simulink model "psm_mpc_ekf_bemf_ctrl"  (R2026a)
settings: Solver=ode23tb  StopTime=simlength  FixedStep=tc  MaxStep=tc
values from neighbouring files (symbols this model uses):
  dead_time_INV = 3e-6    (= 3e-06)    [init_model.m]
  fPWM_INV = fPWM_AFE    (= 15000)    [init_model.m]
  g0_10Hz = fcut_10Hz_flt * ts_afe * 2*pi    (= 0.00418879020479)    [init_model.m]
  g0_1Hz = fcut_1Hz_flt * ts_afe * 2*pi    (= 0.000418879020479)    [init_model.m]
  g1_10Hz = 1 - g0_10Hz    (= 0.995811209795)    [init_model.m]
  g1_1Hz = 1 - g0_1Hz    (= 0.99958112098)    [init_model.m]
  inv_m_scale = motorc_m_scale    [init_model.m]
  iq_lim = 1.4    [init_model.m]
  k_kalman = 0    [init_model.m]
  kg = Kobs(1)    [init_model.m]
  ki_align = 0.1    [init_model.m]
  ki_w = 32    [init_model.m]
  kp_align = 0.6    [init_model.m]
  kp_w = 2    [init_model.m]
  kw = Kobs(2)    [init_model.m]
  lim_down_align = -0.2    [init_model.m]
  lim_up_align = 0.2    [init_model.m]
  number_of_modules = 1    [init_model.m]
  omega_m_sim = omega_m_bez    [init_model.m]
  simlength = 2    [init_model.m]
  tc = ts_afe/100    (= 6.66666666667e-07)    [init_model.m]
  time_gain_afe_module_1 = 1.0    (= 1)    [init_model.m]
  time_gain_inv_module_2 = 1.0    (= 1)    [init_model.m]
  ts_inv = 1/fPWM_INV    (= 6.66666666667e-05)    [init_model.m]
undefined symbols (not defined in the file or in its folder): A1_tilde_ekf, A2_tilde_ekf, A3_tilde_ekf, A4_tilde_ekf, Bd_ekf, C_ekf, ibez, La, Lalpha_norm, Lb, Lbeta_norm, omega_bez, omega_m_bez, psi_bez, psi_m, Qkalman, Rkalman, rpm_base, rpm_bez, Rs, Rs_norm, tau_bez, torque_base, ubez
libraries: fl_lib x24, nesl_utility x11, cstblocks_lti x2, single_phase_pwm_modulator x1, threephase_inductor_lib x1, simple_flexible_shaft x1, permanent_magnet_synchronous_machine x1
(part 2 of 2)

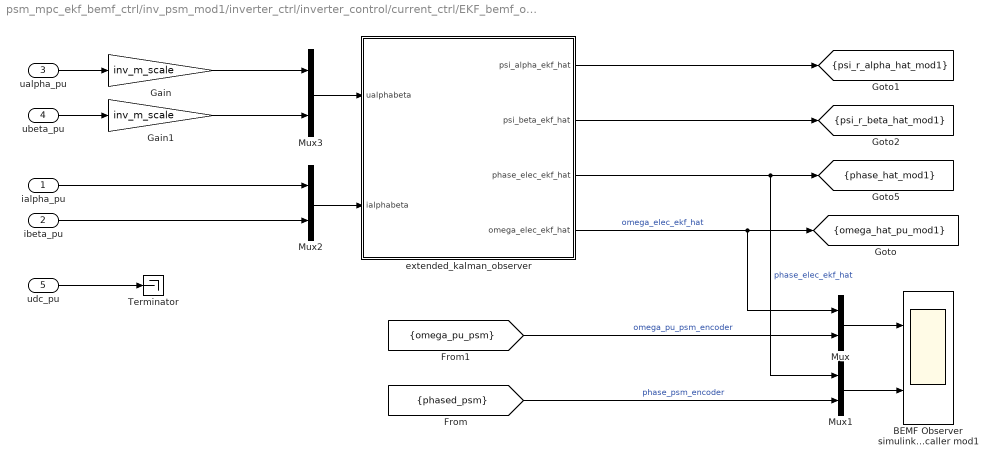
== system psm_mpc_ekf_bemf_ctrl/inv_psm_mod1/inverter_ctrl/inverter_control/current_ctrl/EKF_bemf_observer ==
  ialpha_pu : Inport
  ibeta_pu : Inport  Port=2
  ualpha_pu : Inport  Port=3
  ubeta_pu : Inport  Port=4
  udc_pu : Inport  Port=5
  BEMF Observer simulink/Ccaller mod1 : Scope  NumInputPorts=2
      settings: ActiveDisplayYMinimum=-3.92694091796875  ActiveDisplayYMaximum=3.92645263671875
  Gain : Gain  Gain=inv_m_scale
  Gain1 : Gain  Gain=inv_m_scale
  Mux{,1..3} (4 alike) : Mux  Inputs=2
  Terminator : Terminator
  extended_kalman_observer : Subsystem
  tag scope: omega_hat_pu_mod1=scoped, phase_hat_mod1=scoped, psi_r_alpha_hat_mod1=scoped, psi_r_beta_hat_mod1=scoped
  wires:
  ialpha_pu/1 -> Mux2/1
  ibeta_pu/1 -> Mux2/2
  Mux/1 -> BEMF Observer simulink/Ccaller mod1/1
  Mux1/1 -> BEMF Observer simulink/Ccaller mod1/2
  ualpha_pu/1 -> Gain/1
  ubeta_pu/1 -> Gain1/1
  extended_kalman_observer/3(phase_elec_ekf_hat) -> Mux1/1, [phase_hat_mod1]  "phase_elec_ekf_hat"
  extended_kalman_observer/4(omega_elec_ekf_hat) -> [omega_hat_pu_mod1], Mux/1  "omega_elec_ekf_hat"
  [omega_pu_psm] -> Mux/2  "omega_pu_psm_encoder"
  [phased_psm] -> Mux1/2  "phase_psm_encoder"
  udc_pu/1 -> Terminator/1
  extended_kalman_observer/1(psi_alpha_ekf_hat) -> [psi_r_alpha_hat_mod1]
  extended_kalman_observer/2(psi_beta_ekf_hat) -> [psi_r_beta_hat_mod1]
  Mux2/1 -> extended_kalman_observer/2(ialphabeta)
  Mux3/1 -> extended_kalman_observer/1(ualphabeta)
  Gain/1 -> Mux3/1
  Gain1/1 -> Mux3/2

== system psm_mpc_ekf_bemf_ctrl/inv_psm_mod1/inverter_ctrl/inverter_control/current_ctrl/current_reference_generator ==
  torque_ref_pu : Inport
  theta_elec_hat : Inport  Port=2
  Gain5 : Gain  Gain=-1
  Product : Product
  Product1 : Product
  Trigonometric Function1 : Trigonometry
  Trigonometric Function2 : Trigonometry  Operator=cos
  i_alpha_ref : Outport
  i_beta_ref : Outport  Port=2
  tag scope: ialpha_pu_ref_mod1=scoped, ibeta_pu_ref_mod1=scoped
  wires:
  Trigonometric Function1/1 -> Product/2
  Product1/1 -> [ibeta_pu_ref_mod1], i_beta_ref/1
  Trigonometric Function2/1 -> Product1/2
  Product/1 -> Gain5/1
  Gain5/1 -> [ialpha_pu_ref_mod1], i_alpha_ref/1
  torque_ref_pu/1 -> Product/1, Product1/1
  theta_elec_hat/1 -> Trigonometric Function1/1, Trigonometric Function2/1  "theta_electrical"

== system psm_mpc_ekf_bemf_ctrl/inv_psm_mod1/inverter_ctrl/inverter_control/current_ctrl/current_transformation ==
  Demux : Demux  Outputs=3
  alphabeta2dq : MATLAB Function  TreatAsAtomicUnit=on
  uvw2alphabeta : MATLAB Function  TreatAsAtomicUnit=on
  tag scope: ialpha_pu_mod1=scoped, ibeta_pu_mod1=scoped, id_pu_mod1=scoped, iq_pu_mod1=scoped
  wires:
  alphabeta2dq/2(q) -> [iq_pu_mod1]  "iq_pu"
  alphabeta2dq/1(d) -> [id_pu_mod1]  "id_pu"
  uvw2alphabeta/2(beta) -> alphabeta2dq/2(beta), [ibeta_pu_mod1]  "ibeta_pu"
  uvw2alphabeta/1(alpha) -> [ialpha_pu_mod1], alphabeta2dq/1(alpha)  "ialpha_pu"
  [motor_phase_ctrl_mod1] -> alphabeta2dq/3(gamma)
  Demux/3 -> uvw2alphabeta/3(w)  "iw"
  Demux/2 -> uvw2alphabeta/2(v)  "iv"
  Demux/1 -> uvw2alphabeta/1(u)  "iu"
  [isd_uvw_inv_mod1] -> Demux/1

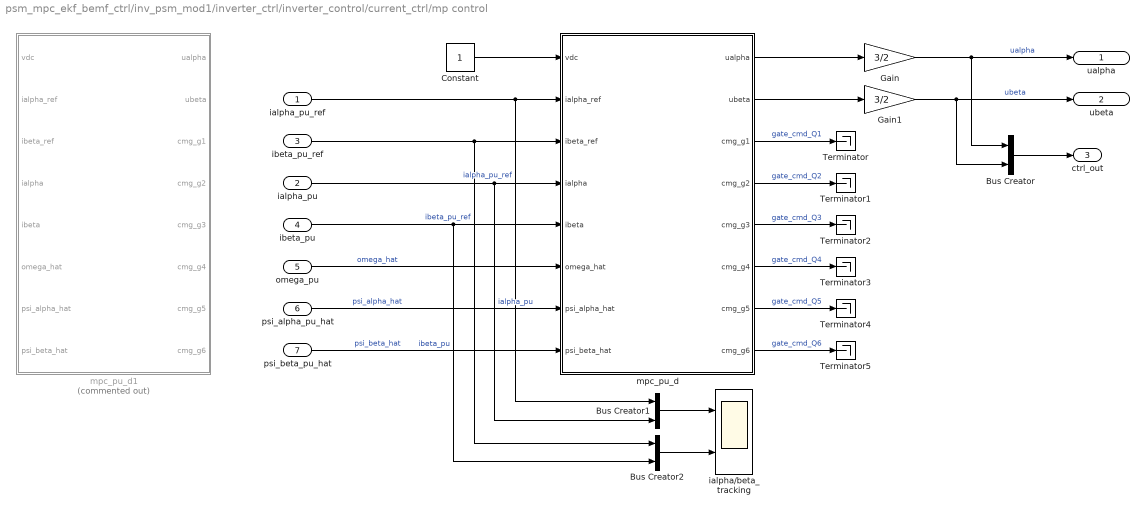
== system psm_mpc_ekf_bemf_ctrl/inv_psm_mod1/inverter_ctrl/inverter_control/current_ctrl/mp control ==
  ialpha_pu_ref : Inport
  ialpha_pu : Inport  Port=2
  ibeta_pu_ref : Inport  Port=3
  ibeta_pu : Inport  Port=4
  omega_pu : Inport  Port=5
  psi_alpha_pu_hat : Inport  Port=6
  psi_beta_pu_hat : Inport  Port=7
  Bus Creator : BusCreator  Inputs=2
  Bus Creator1 : BusCreator  Inputs=2
  Bus Creator2 : BusCreator  Inputs=2
  Constant : Constant
  Gain : Gain  Gain=3/2
  Gain1 : Gain  Gain=3/2
  Terminator{,1..5} (6 alike) : Terminator
  ialpha/beta_tracking : Scope  NumInputPorts=2
      settings: ActiveDisplayYMinimum=-1.13592529296875  ActiveDisplayYMaximum=1.13153076171875  DataLoggingVariableName=ScopeData2
  mpc_pu_d : MATLAB Function  TreatAsAtomicUnit=on
  mpc_pu_d1 : MATLAB Function  Commented=on  TreatAsAtomicUnit=on
  ualpha : Outport
  ubeta : Outport  Port=2
  ctrl_out : Outport  Port=3
  wires:
  ialpha_pu_ref/1 -> mpc_pu_d/2(ialpha_ref), Bus Creator1/1  "ialpha_pu_ref"
  ibeta_pu_ref/1 -> mpc_pu_d/3(ibeta_ref), Bus Creator2/1  "ibeta_pu_ref"
  ialpha_pu/1 -> mpc_pu_d/4(ialpha), Bus Creator1/2  "ialpha_pu"
  ibeta_pu/1 -> mpc_pu_d/5(ibeta), Bus Creator2/2  "ibeta_pu"
  omega_pu/1 -> mpc_pu_d/6(omega_hat)  "omega_hat"
  psi_alpha_pu_hat/1 -> mpc_pu_d/7(psi_alpha_hat)  "psi_alpha_hat"
  psi_beta_pu_hat/1 -> mpc_pu_d/8(psi_beta_hat)  "psi_beta_hat"
  Constant/1 -> mpc_pu_d/1(vdc)
  Bus Creator1/1 -> ialpha/beta_tracking/1
  Bus Creator2/1 -> ialpha/beta_tracking/2
  Bus Creator/1 -> ctrl_out/1
  mpc_pu_d/1(ualpha) -> Gain/1
  mpc_pu_d/2(ubeta) -> Gain1/1
  mpc_pu_d/3(cmg_g1) -> Terminator/1  "gate_cmd_Q1"
  mpc_pu_d/4(cmg_g2) -> Terminator1/1  "gate_cmd_Q2"
  mpc_pu_d/5(cmg_g3) -> Terminator2/1  "gate_cmd_Q3"
  mpc_pu_d/6(cmg_g4) -> Terminator3/1  "gate_cmd_Q4"
  mpc_pu_d/7(cmg_g5) -> Terminator4/1  "gate_cmd_Q5"
  mpc_pu_d/8(cmg_g6) -> Terminator5/1  "gate_cmd_Q6"
  Gain/1 -> Bus Creator/1, ualpha/1  "ualpha"
  Gain1/1 -> Bus Creator/2, ubeta/1  "ubeta"

== system psm_mpc_ekf_bemf_ctrl/inv_psm_mod1/inverter_ctrl/inverter_control/encoder-sensorless-switch/double_integrator_observer ==
  phase_psm : Inport
  Dead Zone : DeadZone  LowerValue=-0.01  UpperValue=0.01
  Gain : Gain  Gain=kw
  Gain1 : Gain  Gain=kg
  Gain2 : Gain  Gain=omega_bez
  Gain3 : Gain  Gain=1/omega_bez
  Gain5 : Gain  Gain=ts_inv
  Sum : Sum  Inputs=-+|
  Sum1 : Sum  Inputs=|++
  Sum2 : Sum  Inputs=|++
  Sum8 : Sum  Inputs=++|
  Unit Delay1 : UnitDelay  InitialCondition=pi  SampleTime=-1
  Unit Delay2 : UnitDelay  SampleTime=-1
  bounder1 : MATLAB Function  TreatAsAtomicUnit=on
  bounder2 : MATLAB Function  TreatAsAtomicUnit=on
  phase_psm_hat : Outport  VectorParamsAs1DForOutWhenUnconnected=off
  omega_pu_psm_hat : Outport  Port=2  VectorParamsAs1DForOutWhenUnconnected=off
  wires:
  Gain1/1 -> Sum2/1
  phase_psm/1 -> Sum/2
  Sum8/1 -> Unit Delay1/1
  Unit Delay1/1 -> bounder2/1(u)
  Sum1/1 -> Unit Delay2/1
  Gain/1 -> Gain3/1
  Unit Delay2/1 -> omega_pu_psm_hat/1, Sum1/2, Gain5/1
  Sum2/1 -> Sum8/2
  bounder2/1(y) -> Sum2/2, phase_psm_hat/1, Sum/1  "phase_hat"
  bounder1/1(y) -> Gain1/1, Gain/1
  Gain2/1 -> Sum8/1
  Gain3/1 -> Sum1/1
  Gain5/1 -> Gain2/1
  Sum/1 -> bounder1/1(u)

== system psm_mpc_ekf_bemf_ctrl/inv_psm_mod1/inverter_ctrl/inverter_control/is inv quantizzation and one step delay/is inv quantizzation and one step delay ==
  is_u_pu : Inport
  is_v_pu : Inport  Port=2
  is_w_pu : Inport  Port=3
  Gain3 : Gain  Gain=-1
  Gain4 : Gain  Gain=-1
  Gain5 : Gain  Gain=-1
  Quantizer : Quantizer  QuantizationInterval=adc_quantization
  Quantizer1 : Quantizer  QuantizationInterval=adc_quantization
  Quantizer2 : Quantizer  QuantizationInterval=adc_quantization
  Unit Delay : UnitDelay  SampleTime=-1
  Unit Delay1 : UnitDelay  SampleTime=-1
  Unit Delay2 : UnitDelay  SampleTime=-1
  Zero-Order Hold : ZeroOrderHold  SampleTime=-1
  Zero-Order Hold1 : ZeroOrderHold  SampleTime=-1
  Zero-Order Hold2 : ZeroOrderHold  SampleTime=-1
  isd_u_pu : Outport
  isd_v_pu : Outport  Port=2
  isd_w_pu : Outport  Port=3
  wires:
  Unit Delay/1 -> Gain3/1
  Unit Delay1/1 -> Gain4/1
  Unit Delay2/1 -> Gain5/1
  Quantizer/1 -> Unit Delay/1
  Quantizer1/1 -> Unit Delay1/1
  Quantizer2/1 -> Unit Delay2/1
  is_u_pu/1 -> Zero-Order Hold/1
  is_v_pu/1 -> Zero-Order Hold1/1
  is_w_pu/1 -> Zero-Order Hold2/1
  Gain3/1 -> isd_u_pu/1
  Gain4/1 -> isd_v_pu/1
  Gain5/1 -> isd_w_pu/1
  Zero-Order Hold/1 -> Quantizer/1
  Zero-Order Hold1/1 -> Quantizer1/1
  Zero-Order Hold2/1 -> Quantizer2/1

== system psm_mpc_ekf_bemf_ctrl/inv_psm_mod1/inverter_ctrl/inverter_control/omega_pu/flt ==
  input : Inport
  Gain3 : Gain  Gain=g1_10Hz
  Gain6 : Gain  Gain=g0_10Hz
  Sum : Sum  Inputs=|++
  Unit Delay1 : UnitDelay  SampleTime=-1
  output : Outport  VectorParamsAs1DForOutWhenUnconnected=off
  wires:
  Gain6/1 -> Sum/1
  input/1 -> Gain6/1
  Unit Delay1/1 -> Gain3/1
  Gain3/1 -> Sum/2
  Sum/1 -> Unit Delay1/1, output/1

== system psm_mpc_ekf_bemf_ctrl/inv_psm_mod1/inverter_ctrl/inverter_control/phase_compensation_1/alignment_ctrl ==
  local_time : Inport
  master_time : Inport  Port=2
  Constant : Constant  Value=0
  Gain : Gain  Gain=-1
  Sum : Sum  Inputs=|+-
  pi : Subsystem  mask{kp=kp_align, ki=ki_align, lim_up=lim_up_align, lim_down=lim_down_align}
      mask prompts: ki "ki*ts"
      mask Display:
      | disp('pi()');
      | port_label('input', 1, 'u_ref');
      | port_label('input', 2, 'u');
      | port_label('output', 1, 'y');
  dp : Outport
  wires:
  master_time/1 -> Sum/1
  Sum/1 -> Gain/1
  Constant/1 -> pi/1(u_ref)
  local_time/1 -> Sum/2
  Gain/1 -> pi/2(u)
  pi/1(y) -> dp/1

== system psm_mpc_ekf_bemf_ctrl/inv_psm_mod1/inverter_ctrl/inverter_control/speed_reference_generator/flt ==
  input : Inport
  Gain3 : Gain  Gain=g1_1Hz
  Gain6 : Gain  Gain=g0_1Hz
  Sum : Sum  Inputs=|++
  Unit Delay1 : UnitDelay  SampleTime=-1
  output : Outport  VectorParamsAs1DForOutWhenUnconnected=off
  wires:
  Gain6/1 -> Sum/1
  input/1 -> Gain6/1
  Unit Delay1/1 -> Gain3/1
  Gain3/1 -> Sum/2
  Sum/1 -> Unit Delay1/1, output/1

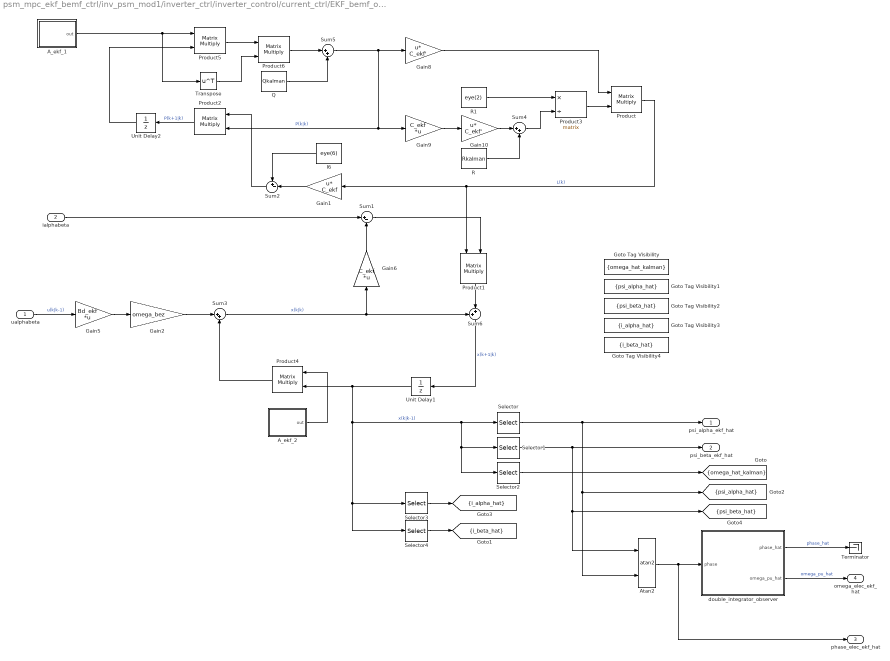
== system psm_mpc_ekf_bemf_ctrl/inv_psm_mod1/inverter_ctrl/inverter_control/current_ctrl/EKF_bemf_observer/extended_kalman_observer ==
  ualphabeta : Inport
  ialphabeta : Inport  Port=2
  A_ekf_1 : Subsystem
  A_ekf_2 : Subsystem
  Atan2 : Trigonometry  Operator=atan2
  Gain1 : Gain  Gain=C_ekf  Multiplication=Matrix(u*K)
  Gain10 : Gain  Gain=C_ekf'  Multiplication=Matrix(u*K)
  Gain2 : Gain  Gain=omega_bez
  Gain5 : Gain  Gain=Bd_ekf  Multiplication=Matrix(K*u)
  Gain6 : Gain  Gain=C_ekf  Multiplication=Matrix(K*u)
  Gain8 : Gain  Gain=C_ekf'  Multiplication=Matrix(u*K)
  Gain9 : Gain  Gain=C_ekf  Multiplication=Matrix(K*u)
  Goto Tag Visibility : GotoTagVisibility  GotoTag=omega_hat_kalman
  Goto Tag Visibility1 : GotoTagVisibility  GotoTag=psi_alpha_hat
  Goto Tag Visibility2 : GotoTagVisibility  GotoTag=psi_beta_hat
  Goto Tag Visibility3 : GotoTagVisibility  GotoTag=i_alpha_hat
  Goto Tag Visibility4 : GotoTagVisibility  GotoTag=i_beta_hat
  I6 : Constant  Value=eye(6)
  Product{,1..2,4..6} (6 alike) : Product  Multiplication=Matrix(*)
  Product3 : Product  Inputs=*/  Multiplication=Matrix(*)
  Q : Constant  Value=Qkalman
  R : Constant  Value=Rkalman
  R1 : Constant  Value=eye(2)
  Selector : Selector  InputPortWidth=6  IndexOptions=Index vector (dialog)  Indices=3  OutputSizes=1
  Selector1 : Selector  InputPortWidth=6  IndexOptions=Index vector (dialog)  Indices=4  OutputSizes=1
  Selector2 : Selector  InputPortWidth=6  IndexOptions=Index vector (dialog)  Indices=6  OutputSizes=1
  Selector3 : Selector  InputPortWidth=6  IndexOptions=Index vector (dialog)  Indices=1  OutputSizes=1
  Selector4 : Selector  InputPortWidth=6  IndexOptions=Index vector (dialog)  Indices=2  OutputSizes=1
  Sum1 : Sum  Inputs=|+-
  Sum2 : Sum  Inputs=+-|
  Sum3 : Sum  Inputs=|++
  Sum4 : Sum  Inputs=|++
  Sum5 : Sum  Inputs=|++
  Sum6 : Sum  Inputs=++|
  Terminator : Terminator
  Transpose : Math  Operator=transpose
  Unit Delay1 : UnitDelay  InitialCondition=[0 0 1 1 0 0]*ts_inv  SampleTime=-1
  Unit Delay2 : UnitDelay  SampleTime=-1
  double_integrator_observer : Subsystem
  psi_alpha_ekf_hat : Outport
  psi_beta_ekf_hat : Outport  Port=2
  phase_elec_ekf_hat : Outport  Port=3
  omega_elec_ekf_hat : Outport  Port=4
  tag scope: i_alpha_hat=scoped, i_beta_hat=scoped, omega_hat_kalman=scoped, psi_alpha_hat=scoped, psi_beta_hat=scoped
  wires:
  Gain5/1 -> Gain2/1
  Gain6/1 -> Sum1/2
  Sum5/1 -> Gain8/1, Gain9/1, Product2/2  "P(k|k)"
  Product5/1 -> Product6/1
  Product6/1 -> Sum5/1
  Q/1 -> Sum5/2
  Gain9/1 -> Gain10/1
  R/1 -> Sum4/2
  Gain10/1 -> Sum4/1
  Gain8/1 -> Product/1
  Product/1 -> Product1/1, Gain1/1  "L(k)"
  Product2/1 -> Unit Delay2/1  "P(k+1|k)"
  Sum2/1 -> Product2/1
  Unit Delay2/1 -> Product5/2
  Sum6/1 -> Unit Delay1/1  "x(k+1|k)"
  I6/1 -> Sum2/1
  Gain1/1 -> Sum2/2
  Sum1/1 -> Product1/2
  ialphabeta/1 -> Sum1/1
  Sum4/1 -> Product3/2
  Product3/1 -> Product/2
  R1/1 -> Product3/1
  ualphabeta/1 -> Gain5/1  "u(k|k-1)"
  Sum3/1 -> Gain6/1, Sum6/1  "x(k|k)"
  Unit Delay1/1 -> Selector2/1, Selector1/1, Selector/1, Selector3/1, Selector4/1, Product4/2  "x(k|k-1)"
  A_ekf_2/1(out) -> Product4/1
  A_ekf_1/1(out) -> Transpose/1, Product5/1
  Product1/1 -> Sum6/2
  Selector1/1 -> Atan2/1, [psi_beta_hat], psi_beta_ekf_hat/1
  Selector/1 -> Atan2/2, [psi_alpha_hat], psi_alpha_ekf_hat/1
  Transpose/1 -> Product6/2
  Selector2/1 -> [omega_hat_kalman]
  Selector3/1 -> [i_alpha_hat]
  Selector4/1 -> [i_beta_hat]
  Product4/1 -> Sum3/2
  double_integrator_observer/2(omega_pu_hat) -> omega_elec_ekf_hat/1  "omega_pu_hat"
  Atan2/1 -> double_integrator_observer/1(phase), phase_elec_ekf_hat/1
  double_integrator_observer/1(phase_hat) -> Terminator/1  "phase_hat"
  Gain2/1 -> Sum3/1

== system psm_mpc_ekf_bemf_ctrl/inv_psm_mod1/inverter_ctrl/inverter_control/phase_compensation_1/alignment_ctrl/pi ==
  u_ref : Inport
  u : Inport  Port=2
  1/Ti : Gain  Gain=kp  SaturateOnIntegerOverflow=on  OutDataTypeStr=Inherit: Same as input  ParamDataTypeStr=Inherit: Same as input
  Saturation : Saturate  UpperLimit=lim_up  LowerLimit=lim_down
  Sum1 : Sum  Inputs=+++  SaturateOnIntegerOverflow=on
  Sum2 : Sum  Inputs=-+  SaturateOnIntegerOverflow=on
  Sum3 : Sum  Inputs=-+  SaturateOnIntegerOverflow=on
  Unit Delay4 : UnitDelay  SampleTime=-1
  kp : Gain  Gain=ki  SaturateOnIntegerOverflow=on  OutDataTypeStr=Inherit: Same as input  ParamDataTypeStr=Inherit: Same as input
  y : Outport
  wires:
  1/Ti/1 -> Sum1/1, Sum3/1
  kp/1 -> Sum1/2
  Sum3/1 -> Unit Delay4/1
  Unit Delay4/1 -> Sum1/3
  u_ref/1 -> Sum2/2
  u/1 -> Sum2/1
  Sum2/1 -> kp/1, 1/Ti/1
  Sum1/1 -> Saturation/1
  Saturation/1 -> Sum3/2, y/1

== system psm_mpc_ekf_bemf_ctrl/inv_psm_mod1/inverter_ctrl/inverter_control/current_ctrl/EKF_bemf_observer/extended_kalman_observer/A_ekf_1 ==
  Gain1 : Gain  Gain=A2_tilde_ekf
  Gain{7..10} (4 alike) : Gain  Gain=omega_bez
  Gain{2,4,6,11} (4 alike) : Gain  Gain=ts_inv
  Gain3 : Gain  Gain=A3_tilde_ekf
  Gain5 : Gain  Gain=A4_tilde_ekf
  I1 : Constant  Value=eye(6)
  I2 : Constant  Value=A1_tilde_ekf
  Sum7 : Sum  Inputs=+++++
  out : Outport
  wires:
  [psi_beta_hat] -> Gain5/1
  [psi_alpha_hat] -> Gain3/1
  [omega_hat_kalman] -> Gain1/1
  Gain5/1 -> Gain6/1
  Gain3/1 -> Gain4/1
  Gain1/1 -> Gain2/1
  I1/1 -> Sum7/1
  I2/1 -> Gain11/1
  Sum7/1 -> out/1
  Gain11/1 -> Gain7/1
  Gain2/1 -> Gain8/1
  Gain4/1 -> Gain9/1
  Gain6/1 -> Gain10/1
  Gain7/1 -> Sum7/2
  Gain8/1 -> Sum7/3
  Gain9/1 -> Sum7/4
  Gain10/1 -> Sum7/5

== system psm_mpc_ekf_bemf_ctrl/inv_psm_mod1/inverter_ctrl/inverter_control/current_ctrl/EKF_bemf_observer/extended_kalman_observer/A_ekf_2 ==
  Gain1 : Gain  Gain=A2_tilde_ekf
  Gain{7..10} (4 alike) : Gain  Gain=omega_bez
  Gain{2,4,6,11} (4 alike) : Gain  Gain=ts_inv
  Gain3 : Gain  Gain=A3_tilde_ekf
  Gain5 : Gain  Gain=A4_tilde_ekf
  I1 : Constant  Value=eye(6)
  I2 : Constant  Value=A1_tilde_ekf
  Sum7 : Sum  Inputs=+++++
  out : Outport
  wires:
  Sum7/1 -> out/1
  I2/1 -> Gain11/1
  I1/1 -> Sum7/1
  Gain1/1 -> Gain2/1
  Gain3/1 -> Gain4/1
  Gain5/1 -> Gain6/1
  [omega_hat_kalman] -> Gain1/1
  [psi_alpha_hat] -> Gain3/1
  [psi_beta_hat] -> Gain5/1
  Gain11/1 -> Gain7/1
  Gain2/1 -> Gain8/1
  Gain4/1 -> Gain9/1
  Gain6/1 -> Gain10/1
  Gain7/1 -> Sum7/2
  Gain8/1 -> Sum7/3
  Gain9/1 -> Sum7/4
  Gain10/1 -> Sum7/5

== system psm_mpc_ekf_bemf_ctrl/inv_psm_mod1/inverter_ctrl/inverter_control/current_ctrl/EKF_bemf_observer/extended_kalman_observer/double_integrator_observer ==
  phase : Inport
  Dead Zone : DeadZone  LowerValue=-0.01  UpperValue=0.01
  Gain : Gain  Gain=kw
  Gain1 : Gain  Gain=kg
  Gain2 : Gain  Gain=omega_bez
  Gain3 : Gain  Gain=1/omega_bez
  Gain5 : Gain  Gain=ts_inv
  Sum : Sum  Inputs=-+|
  Sum1 : Sum  Inputs=|++
  Sum2 : Sum  Inputs=|++
  Sum8 : Sum  Inputs=++|
  Unit Delay1 : UnitDelay  InitialCondition=pi  SampleTime=-1
  Unit Delay2 : UnitDelay  SampleTime=-1
  bounder1 : MATLAB Function  TreatAsAtomicUnit=on
  bounder2 : MATLAB Function  TreatAsAtomicUnit=on
  phase_hat : Outport  VectorParamsAs1DForOutWhenUnconnected=off
  omega_pu_hat : Outport  Port=2  VectorParamsAs1DForOutWhenUnconnected=off
  wires:
  Gain1/1 -> Sum2/1
  phase/1 -> Sum/2
  Sum8/1 -> Unit Delay1/1
  Unit Delay1/1 -> bounder2/1(u)
  Sum1/1 -> Unit Delay2/1
  Gain/1 -> Gain3/1
  Unit Delay2/1 -> omega_pu_hat/1, Sum1/2, Gain5/1
  Sum2/1 -> Sum8/2
  bounder2/1(y) -> Sum2/2, phase_hat/1, Sum/1  "phase_hat"
  bounder1/1(y) -> Gain1/1, Gain/1
  Gain2/1 -> Sum8/1
  Gain3/1 -> Sum1/1
  Gain5/1 -> Gain2/1
  Sum/1 -> bounder1/1(u)

== matlab function psm_mpc_ekf_bemf_ctrl/inv_psm_mod1/inverter_ctrl/inverter_control/current_ctrl/current_transformation/uvw2alphabeta ==
  data: u input; alpha output; v input; w input; beta output
function [alpha,beta] = uvw2alphabeta(u,v,w)

alpha = 2/3*(u - 1/2*v - 1/2*w);
beta  = 2/3*(sqrt(3)/2*(v - w));

end

== matlab function psm_mpc_ekf_bemf_ctrl/inv_psm_mod1/inverter_ctrl/inverter_control/current_ctrl/mp control/mpc_pu_d ==
  data: vdc input; ialpha_ref input; ibeta_ref input; ialpha input; ualpha output; ibeta input; omega_hat input; psi_alpha_hat input; psi_beta_hat input; ubeta output; cmg_g1 output; cmg_g2 output; cmg_g3 output; cmg_g4 output; cmg_g5 output; cmg_g6 output; Rs_norm parameter; Lalpha_norm parameter; Lbeta_norm parameter; ts_inv parameter; k_kalman parameter; omega_bez parameter
function [ualpha, ubeta, cmg_g1, cmg_g2, cmg_g3, cmg_g4, cmg_g5, cmg_g6] = ...
    mpc(vdc, ialpha_ref, ibeta_ref, ialpha, ibeta, omega_hat, ...
        psi_alpha_hat, psi_beta_hat, Rs_norm, Lalpha_norm, Lbeta_norm, ...
        ts_inv, k_kalman, omega_bez)

    persistent ualpha_z ubeta_z

    % ------------------------------------------------------------------ %
    %  Voltage vectors in alpha-beta frame  (index 0..6, row = vector)   %
    %  Row order: [u0, u1, u2, u3, u4, u5, u6]                           %
    % ------------------------------------------------------------------ %
    k = 2/3 * vdc;
    UV = k * [  0,          0        ;   % u0  (zero)
                1,          0        ;   % u1
                1/2,        sqrt(3)/2;   % u2
               -1/2,        sqrt(3)/2;   % u3
               -1,          0        ;   % u4
               -1/2,       -sqrt(3)/2;   % u5
                1/2,       -sqrt(3)/2 ]; % u6

    % Gate patterns [g1 g2 g3 g4 g5 g6] for each vector (on=15, off=0)
    on = 15; off = 0;
    GATES = [ on, off, on,  off, on,  off;   % u0
              on, off, off, on,  off, on ;   % u1
              on, off, on,  off, off, on ;   % u2
              off, on, on,  off, off, on ;   % u3
              off, on, on,  off, on,  off;   % u4
              off, on, off, on,  on,  off;   % u5
              on,  off, off, on,  on,  off]; % u6

    % Admissible next vectors given current vector (switching constraint)
    % zero vector can go anywhere; active vector -> zero + two adjacent
    ADMIT = { 1:7;           % from u0: all 7
              [1, 2, 7];     % from u1: u0, u1, u6
              [1, 2, 3];     % from u2: u0, u1, u2  -- NB: was u1,u2,u3 in original
              [1, 3, 4];     % from u3: u0, u2, u3
              [1, 4, 5];     % from u4: u0, u3, u4
              [1, 5, 6];     % from u5: u0, u4, u5
              [1, 6, 7] };   % from u6: u0, u5, u6

    % ------------------------------------------------------------------ %
    %  Initialise persistent state                                        %
    % ------------------------------------------------------------------ %
    if isempty(ualpha_z)
        ualpha_z = 0;
        ubeta_z  = 0;
    end

    % ------------------------------------------------------------------ %
    %  Common terms (factor out repeated computation)                     %
    % ------------------------------------------------------------------ %
    ts = ts_inv * omega_bez;

    ia_common = (1 - Rs_norm/Lalpha_norm*ts)*ialpha + omega_hat/Lalpha_norm*psi_beta_hat*ts;
    ib_common = (1 - Rs_norm/Lbeta_norm *ts)*ibeta  - omega_hat/Lbeta_norm *psi_alpha_hat*ts;

    % Predicted currents for ALL 7 vectors (7x2 matrix)
    ia_pred = ia_common + UV(:,1) * (ts/Lalpha_norm);   % 7x1
    ib_pred = ib_common + UV(:,2) * (ts/Lbeta_norm );   % 7x1

    % Cost function for all vectors (7x1)
    J = (ialpha_ref - ia_pred).^2 + (ibeta_ref - ib_pred).^2 ...
      + k_kalman * (UV(:,1).^2 + UV(:,2).^2);

    % ------------------------------------------------------------------ %
    %  Switching constraint: find index of current vector (1-based)       %
    % ------------------------------------------------------------------ %
    [~, prev_idx] = ismember([ualpha_z, ubeta_z], UV, 'rows');
    if prev_idx == 0, prev_idx = 1; end   % fallback to u0

    % Restrict search to admissible candidates
    candidates = ADMIT{prev_idx};
    [~, best_local] = min(J(candidates));
    best_idx = candidates(best_local);

    ualpha = UV(best_idx, 1);
    ubeta  = UV(best_idx, 2);

    ualpha_z = ualpha;
    ubeta_z  = ubeta;

    % ------------------------------------------------------------------ %
    %  Gate signals                                                       %
    % ------------------------------------------------------------------ %
    g = GATES(best_idx, :);
    cmg_g1 = g(1); cmg_g2 = g(2); cmg_g3 = g(3);
    cmg_g4 = g(4); cmg_g5 = g(5); cmg_g6 = g(6);
end

== matlab function psm_mpc_ekf_bemf_ctrl/inv_psm_mod1/inverter/timer/MATLAB Function ==
  data: t input; y output; phase input; period input
function y = ramp_up_down(t,phase,period)
x = sin(2*pi/period*t - phase -pi/2);
y = asin(x)/pi + 1/2;

== matlab function psm_mpc_ekf_bemf_ctrl/inv_psm_mod1/inverter_ctrl/inverter_control/encoder-sensorless-switch/double_integrator_observer/bounder1 ==
  data: u input; y output
function y = bounder(u)
    y = -pi + mod(u+3*pi,2*pi);
end

== matlab function psm_mpc_ekf_bemf_ctrl/inv_psm_mod1/inverter_ctrl/inverter_control/encoder-sensorless-switch/double_integrator_observer/bounder2 ==
  data: u input; y output
function y = bounder(u)
    y = -pi + mod(u+3*pi,2*pi);
end

== matlab function psm_mpc_ekf_bemf_ctrl/inv_psm_mod1/inverter_ctrl/inverter_control/current_ctrl/EKF_bemf_observer/extended_kalman_observer/double_integrator_observer/bounder1 ==
  data: u input; y output
function y = bounder(u)
    y = -pi + mod(u+3*pi,2*pi);
end

== matlab function psm_mpc_ekf_bemf_ctrl/inv_psm_mod1/inverter/MATLAB Function ==
  data: ua input; uu output; uv output; uw output; ub input
function [uu, uv, uw] = ab2uvw(ua, ub)

uu = ua;
uv = -ua/2 + sqrt(3)/2*ub;
uw = -ua/2 - sqrt(3)/2*ub;

== matlab function psm_mpc_ekf_bemf_ctrl/inv_psm_mod1/inverter_ctrl/inverter_control/encoder-sensorless-switch/MATLAB Function ==
  data: omega_ctrl output; phase_psm input; omega_obs input; phase_obs input; phase_ctrl output; omega_psm input; omega_th parameter
function [omega_ctrl, phase_ctrl] = switch_enc2obs(phase_psm, omega_obs, phase_obs, omega_psm, omega_th)

if abs(omega_psm) > omega_th
    omega_ctrl = omega_obs;
    phase_ctrl = phase_obs;
else
    omega_ctrl = omega_psm;
    phase_ctrl = phase_psm;
end

== matlab function psm_mpc_ekf_bemf_ctrl/inv_psm_mod1/inverter_ctrl/inverter_control/current_ctrl/EKF_bemf_observer/extended_kalman_observer/double_integrator_observer/bounder2 ==
  data: u input; y output
function y = bounder(u)
    y = -pi + mod(u+3*pi,2*pi);
end

== matlab function psm_mpc_ekf_bemf_ctrl/inv_psm_mod1/inverter_ctrl/inverter_control/current_ctrl/current_transformation/alphabeta2dq ==
  data: alpha input; d output; beta input; gamma input; q output
function [d,q] = alphabeta2dq(alpha,beta,gamma)

    d  =  alpha*cos(gamma) + beta*sin(gamma);
    q = -alpha*sin(gamma) + beta*cos(gamma);

end

== matlab function psm_mpc_ekf_bemf_ctrl/inv_psm_mod1/inverter_ctrl/inverter_control/current_ctrl/mp control/mpc_pu_d1 ==
  data: vdc input; ialpha_ref input; ibeta_ref input; ialpha input; ualpha output; ibeta input; omega_hat input; psi_alpha_hat input; psi_beta_hat input; ubeta output; cmg_g1 output; cmg_g2 output; cmg_g3 output; cmg_g4 output; cmg_g5 output; cmg_g6 output; Rs_norm parameter; Lalpha_norm parameter; Lbeta_norm parameter; ts_inv parameter; k_kalman parameter; omega_bez parameter
function [ualpha, ubeta, cmg_g1, cmg_g2, cmg_g3, cmg_g4, cmg_g5, cmg_g6]    = mpc(vdc, ialpha_ref,...
    ibeta_ref, ialpha, ibeta, omega_hat, psi_alpha_hat, psi_beta_hat, Rs_norm, Lalpha_norm, Lbeta_norm, ...
    ts_inv, k_kalman, omega_bez)

    persistent ualpha_z ubeta_z

    on = 15;
    off = 0;

    ualpha_1 = 2/3*vdc;
    ubeta_1 = 0;

    ualpha_2 = 2/3*1/2*vdc;
    ubeta_2 = 2/3*sqrt(3)/2*vdc;

    ualpha_3 = -2/3*1/2*vdc;
    ubeta_3 = 2/3*sqrt(3)/2*vdc;

    ualpha_4 = -2/3*vdc;
    ubeta_4 = 0;

    ualpha_5 = -2/3*1/2*vdc;
    ubeta_5 = -2/3*sqrt(3)/2*vdc;

    ualpha_6 = 2/3*1/2*vdc;
    ubeta_6 = -2/3*sqrt(3)/2*vdc;

    ualpha_0 = 0;
    ubeta_0 = 0;

    if isempty(ualpha_z)
        ualpha_z = 0;
        ubeta_z = 0;
    end
    
    ts = ts_inv*omega_bez;

    ia_p0 = (1-Rs_norm/Lalpha_norm*ts)*ialpha + omega_hat/Lalpha_norm*psi_beta_hat*ts + ualpha_0*ts/Lalpha_norm;
    ib_p0 = (1-Rs_norm/Lbeta_norm*ts)*ibeta - omega_hat/Lbeta_norm*psi_alpha_hat*ts + ubeta_0*ts/Lbeta_norm;
    
    ia_p1 = (1-Rs_norm/Lalpha_norm*ts)*ialpha + omega_hat/Lalpha_norm*psi_beta_hat*ts + ualpha_1*ts/Lalpha_norm;
    ib_p1 = (1-Rs_norm/Lbeta_norm*ts)*ibeta - omega_hat/Lbeta_norm*psi_alpha_hat*ts + ubeta_1*ts/Lbeta_norm;

    ia_p2 = (1-Rs_norm/Lalpha_norm*ts)*ialpha + omega_hat/Lalpha_norm*psi_beta_hat*ts + ualpha_2*ts/Lalpha_norm;
    ib_p2 = (1-Rs_norm/Lbeta_norm*ts)*ibeta - omega_hat/Lbeta_norm*psi_alpha_hat*ts + ubeta_2*ts/Lbeta_norm;

    ia_p3 = (1-Rs_norm/Lalpha_norm*ts)*ialpha + omega_hat/Lalpha_norm*psi_beta_hat*ts + ualpha_3*ts/Lalpha_norm;
    ib_p3 = (1-Rs_norm/Lbeta_norm*ts)*ibeta - omega_hat/Lbeta_norm*psi_alpha_hat*ts + ubeta_3*ts/Lbeta_norm;

    ia_p4 = (1-Rs_norm/Lalpha_norm*ts)*ialpha + omega_hat/Lalpha_norm*psi_beta_hat*ts + ualpha_4*ts/Lalpha_norm;
    ib_p4 = (1-Rs_norm/Lbeta_norm*ts)*ibeta - omega_hat/Lbeta_norm*psi_alpha_hat*ts + ubeta_4*ts/Lbeta_norm;

    ia_p5 = (1-Rs_norm/Lalpha_norm*ts)*ialpha + omega_hat/Lalpha_norm*psi_beta_hat*ts + ualpha_5*ts/Lalpha_norm;
    ib_p5 = (1-Rs_norm/Lbeta_norm*ts)*ibeta - omega_hat/Lbeta_norm*psi_alpha_hat*ts + ubeta_5*ts/Lbeta_norm;

    ia_p6 = (1-Rs_norm/Lalpha_norm*ts)*ialpha + omega_hat/Lalpha_norm*psi_beta_hat*ts + ualpha_6*ts/Lalpha_norm;
    ib_p6 = (1-Rs_norm/Lbeta_norm*ts)*ibeta - omega_hat/Lbeta_norm*psi_alpha_hat*ts + ubeta_6*ts/Lbeta_norm;
  
    J0 = (ialpha_ref - ia_p0)^2 + (ibeta_ref - ib_p0)^2 + k_kalman * (ualpha_0^2 + ubeta_0^2);
    J1 = (ialpha_ref - ia_p1)^2 + (ibeta_ref - ib_p1)^2 + k_kalman * (ualpha_1^2 + ubeta_1^2);
    J2 = (ialpha_ref - ia_p2)^2 + (ibeta_ref - ib_p2)^2 + k_kalman * (ualpha_2^2 + ubeta_2^2);
    J3 = (ialpha_ref - ia_p3)^2 + (ibeta_ref - ib_p3)^2 + k_kalman * (ualpha_3^2 + ubeta_3^2);
    J4 = (ialpha_ref - ia_p4)^2 + (ibeta_ref - ib_p4)^2 + k_kalman * (ualpha_4^2 + ubeta_4^2);
    J5 = (ialpha_ref - ia_p5)^2 + (ibeta_ref - ib_p5)^2 + k_kalman * (ualpha_5^2 + ubeta_5^2);
    J6 = (ialpha_ref - ia_p6)^2 + (ibeta_ref - ib_p6)^2 + k_kalman * (ualpha_6^2 + ubeta_6^2);
    
    if (ualpha_z == ualpha_0) && (ubeta_z == ubeta_0)
        [m,i] = min([J0, J1, J2, J3, J4, J5, J6]);
        if i == 1
            ualpha = ualpha_0;
            ubeta = ubeta_0;
        elseif i == 2
            ualpha = ualpha_1;
            ubeta = ubeta_1;
        elseif i == 3
            ualpha = ualpha_2;
            ubeta = ubeta_2;
        elseif i == 4
            ualpha = ualpha_3;
            ubeta = ubeta_3;
        elseif i == 5
            ualpha = ualpha_4;
            ubeta = ubeta_4;
        elseif i == 6
            ualpha = ualpha_5;
            ubeta = ubeta_5;
        else
            ualpha = ualpha_6;
            ubeta = ubeta_6;
        end
    elseif (ualpha_z == ualpha_1) && (ubeta_z == ubeta_1)
        [m,i] = min([J0, J1, J2, J6]);
        if i == 1
            ualpha = ualpha_0;
            ubeta = ubeta_0;
        elseif i == 2
            ualpha = ualpha_1;
            ubeta = ubeta_1;
        elseif i == 3
            ualpha = ualpha_2;
            ubeta = ubeta_2;
        else
            ualpha = ualpha_6;
            ubeta = ubeta_6;
        end
    elseif (ualpha_z == ualpha_2) && (ubeta_z == ubeta_2) % vector u2
        [m,i] = min([J0, J1, J2, J3]);
        if i == 1
            ualpha = ualpha_0;
            ubeta = ubeta_0;
        elseif i == 2
            ualpha = ualpha_1;
            ubeta = ubeta_1;
        elseif i == 3
            ualpha = ualpha_2;
            ubeta = ubeta_2;
        else
            ualpha = ualpha_3;
            ubeta = ubeta_3;
        end
    elseif (ualpha_z == ualpha_3) && (ubeta_z == ubeta_3)
        [m,i] = min([J0, J2, J3, J4]);
        if i == 1
            ualpha = ualpha_0;
            ubeta = ubeta_0;
        elseif i == 2
            ualpha = ualpha_2;
            ubeta = ubeta_2;
        elseif i == 3
            ualpha = ualpha_3;
            ubeta = ubeta_3;
        else
            ualpha = ualpha_4;
            ubeta = ubeta_4;
        end
    elseif (ualpha_z == ualpha_4) && (ubeta_z == ubeta_4)
        [m,i] = min([J0, J3, J4, J5]);
        if i == 1
            ualpha = ualpha_0;
            ubeta = ubeta_0;
        elseif i == 2
            ualpha = ualpha_3;
            ubeta = ubeta_3;
        elseif i == 3
            ualpha = ualpha_4;
            ubeta = ubeta_4;
        else
            ualpha = ualpha_5;
            ubeta = ubeta_5;
        end
    elseif (ualpha_z == ualpha_5) && (ubeta_z == ubeta_5) % u5
        [m,i] = min([J0, J4, J5, J6]);
        if i == 1
            ualpha = ualpha_0;
            ubeta = ubeta_0;
        elseif i == 2
            ualpha = ualpha_4;
            ubeta = ubeta_4;
        elseif i == 3
            ualpha = ualpha_5;
            ubeta = ubeta_5;
        else
            ualpha = ualpha_6;
            ubeta = ubeta_6;
        end
    else
        [m,i] = min([J0, J5, J6, J1]);
        if i == 1
            ualpha = ualpha_0;
            ubeta = ubeta_0;
        elseif i == 2
            ualpha = ualpha_5;
            ubeta = ubeta_5;
        elseif i == 3
            ualpha = ualpha_6;
            ubeta = ubeta_6;
        else
            ualpha = ualpha_1;
            ubeta = ubeta_1;
        end
    end
    ualpha_z = ualpha;
    ubeta_z = ubeta;

    if (ualpha == ualpha_0 && ubeta == ubeta_0)
        cmg_g1 = on;
        cmg_g2 = off;
        cmg_g3 = on;
        cmg_g4 = off;
        cmg_g5 = on;
        cmg_g6 = off;
    elseif (ualpha == ualpha_1 && ubeta == ubeta_1)
        cmg_g1 = on;
        cmg_g2 = off;
        cmg_g3 = off;
        cmg_g4 = on;
        cmg_g5 = off;
        cmg_g6 = on;
    elseif (ualpha == ualpha_2 && ubeta == ubeta_2)
        cmg_g1 = on;
        cmg_g2 = off;
        cmg_g3 = on;
        cmg_g4 = off;
        cmg_g5 = off;
        cmg_g6 = on;
    elseif (ualpha == ualpha_3 && ubeta == ubeta_3)
        cmg_g1 = off;
        cmg_g2 = on;
        cmg_g3 = on;
        cmg_g4 = off;
        cmg_g5 = off;
        cmg_g6 = on;
    elseif (ualpha == ualpha_4 && ubeta == ubeta_4)
        cmg_g1 = off;
        cmg_g2 = on;
        cmg_g3 = on;
        cmg_g4 = off;
        cmg_g5 = on;
        cmg_g6 = off;
    elseif (ualpha == ualpha_5 && ubeta == ubeta_5)
        cmg_g1 = off;
        cmg_g2 = on;
        cmg_g3 = off;
        cmg_g4 = on;
        cmg_g5 = on;
        cmg_g6 = off;
    elseif (ualpha == ualpha_6 && ubeta == ubeta_6)
        cmg_g1 = on;
        cmg_g2 = off;
        cmg_g3 = off;
        cmg_g4 = on;
        cmg_g5 = on;
        cmg_g6 = off;
    else
        cmg_g1 = off;
        cmg_g2 = on;
        cmg_g3 = off;
        cmg_g4 = on;
        cmg_g5 = off;
        cmg_g6 = on;
    end  
end
